simulink model "RotaryPendulum_EV3_SwingUp"  (R2015a)
settings: Solver=ode3  SolverMode=SingleTasking  StartTime=0  StopTime=inf  FixedStep=Ts  RelTol=1e-3
PreLoadFcn:
  | RotaryPendulum_PARAM
InitFcn:
  | simMode = get_param(gcs, 'SimulationMode');
  | if strcmp(simMode, 'external')
  | set_param(gcs,'StopTime', 'Inf');
  | elseif strcmp(simMode, 'normal')
  | set_param(gcs,'StopTime', '10');
  | end
model workspace (MAT data in the model file):
  PulseAmplitude = 200
  Amp = 0
  freq = 0
  Sat = 75
  Ts = 0.008
  threshold = 0.785398163397
  Sig = Simulink.Signal
  Sig.DataType = 'auto'
  Sig.Dimensions = -1
  Sig.DimensionsMode = 'auto'
  Sig.Complexity = 'auto'
  Sig.SampleTime = -1
  Sig.SamplingMode = 'auto'
undefined symbols (not defined in the file): B, C, Center, g, l, m
libraries: simulink x6, legoev3lib x6, simulink_extras x1
settings Model: SimulationMode=external  CovSFcnEnable=off  ExtModeTrigDuration=2  Creator=ngautier  LastModifiedBy=mischak
settings OptimizationCC: EnhancedBackFolding=on  CachingGlobalReferences=on  StrengthReduction=on  OptimizeModelRefInitCode=on  LifeSpan=1
settings DebuggingCC: NonBusSignalsTreatedAsBus=error
settings HardwareCC: ProdLargestAtomicInteger=Long  ProdLargestAtomicFloat=Float  ProdEndianess=LittleEndian  ProdHWDeviceType=ARM Compatible->ARM 9
settings RTWCC: SystemTargetFile=realtime.tlc  GenerateMakefile=off  TemplateMakefile=realtime.tmf  Description=Run on Target Hardware  RTWVerbose=off  IncludeHyperlinkInReport=on
settings ERTTargetCC: CombineOutputUpdateFcns=off  ExtMode=on  ExtModeMexArgs=0 8 9600 30  ERTSrcFileBannerTemplate=realtime_code_template.cgt  ERTHdrFileBannerTemplate=realtime_code_template.cgt  ERTDataSrcFileTemplate=realtime_code_template.cgt  ERTDataHdrFileTemplate=realtime_code_template.cgt  ERTCustomFileTemplate=realtime_file_process.tlc

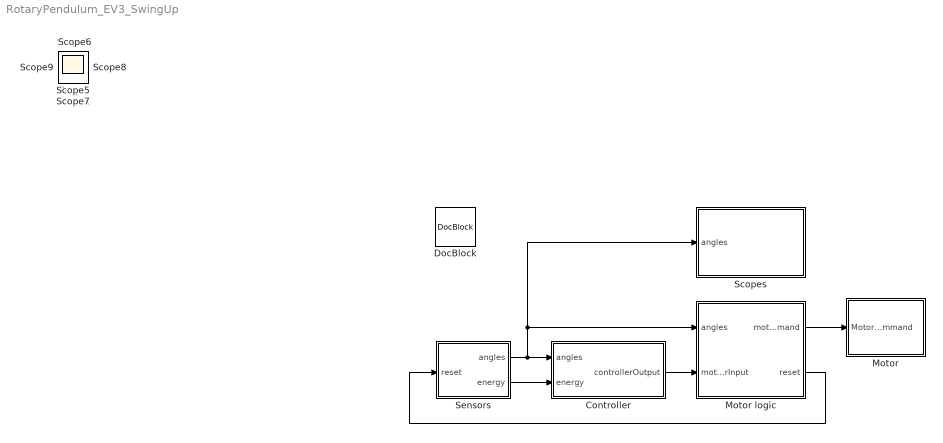
== system RotaryPendulum_EV3_SwingUp ==
  Controller : Subsystem  mask{SUGain=10, outer_gain=[62 9 570 -5], inner_gain=[10 10 370 -10]}
      mask prompts: SUGain "Swing-up amplitude:"; outer_gain "Outer linear gains [al, dal, be, dbe]:"; inner_gain "Inner linear gains [al, dal, be, dbe]:"
      mask TypeOptions SUGain: Swingup controller/Gain
      mask TypeOptions outer_gain: LQR controller/outer_gain
      mask TypeOptions inner_gain: LQR controller/inner_gain
  DocBlock : simulink/Model-Wide Utilities/DocBlock  DocumentType=Text
      content=|
      | Why not use your mobile phone to connect to the EV3?
      |
      | * Enable the portable Wi-Fi hotspot in your mobile phone and note down the
      |   hotspot name and password.
      | * Connect your computer to the hotspot.
      | * Connect the EV3 to the hotspot:
      | ** Navigate to the settings screen (wrench symbol), scroll down and enable [WiFi].
      | ** In the Wi-Fi menu select [Connections] and select the hotspot.
      | ** Enter the hotspot password in [Encryption].
  Motor : Subsystem  mask{sportNumber=C}
      mask prompts: sportNumber "NXT motor port:"
      mask TypeOptions sportNumber: Motor1/sportNumber
      mask Display: image(imread('Motor_icon.jpg'))
  Motor logic : Subsystem  mask{outOfBounds=160}
      mask prompts: outOfBounds "Out of bounds alpha (deg):"
      mask TypeOptions outOfBounds: return&restart/outOfBounds
  Scopes : Subsystem
  Sensors : Subsystem  mask{portNumberAlpha=C, portNumberBeta=B, Value=1}
      mask prompts: portNumberAlpha "NXT alpha sensor port:"; portNumberBeta "NXT beta sensor port:"; Value "Encoder offset (deg):"
      mask TypeOptions portNumberAlpha: Alpha/portNumber
      mask TypeOptions portNumberBeta: Beta/portNumber
      mask TypeOptions Value: Encoder offset/Value
      mask Display: image(imread('Encoders_icon.jpg'))
  Scope{,1..9} (10 alike) : Scope
      Scope1 settings: YMin=3.14159  YMax=3.14159
      Scope2 settings: SaveName=ScopeData2
      Scope3 settings: YMin=3.14159  YMax=3.14159  SaveName=ScopeData3
      Scope4 settings: SaveName=ScopeData4
      Scope5 settings: YMin=0  YMax=0.035  SaveName=ScopeData5
      Scope6 settings: SaveName=ScopeData6
      Scope7 settings: SaveName=ScopeData7
      Scope8 settings: SaveName=ScopeData8
      Scope9 settings: SaveName=ScopeData9
  wires:
  Controller/1(controllerOutput) -> Motor logic/2(motorInput)
  Motor logic/1(motorCommand) -> Motor/1(MotorCommand)
  Sensors/2("energy ") -> Controller/2(energy)
  Sensors/1(angles) -> Motor logic/1(angles), Scopes/1(angles), Controller/1(angles)
  Motor logic/2(reset) -> Sensors/1(reset)

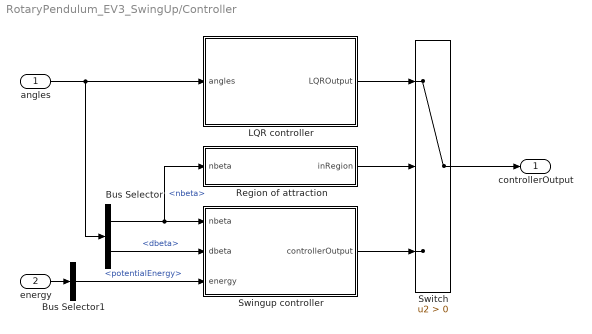
== system RotaryPendulum_EV3_SwingUp/Controller ==
  angles : Inport
  energy : Inport  Port=2
  Bus Selector : BusSelector  OutputSignals=nbeta,dbeta
  Bus Selector1 : BusSelector  OutputSignals=potentialEnergy
  LQR controller : Subsystem  mask{inner_gain=inner_gain, outer_gain=outer_gain}
      mask prompts: inner_gain "Inner gain"; outer_gain "Outer gain"
  Region of attraction : Subsystem  mask{outer_angle=pi/7}
      mask prompts: outer_angle "Simulink:masks:ConstantValue_MP"
      mask TypeOptions outer_angle: Attraction Region/const
      mask Display:
      | %maskValues = get_param(gcb, 'MaskValues');
      | %region = eval(maskValues{1});
      | x = -1:0.1:1;
      | plot(x,abs(x));
      | %ylim([0 2]);
  Swingup controller : Subsystem  SystemSampleTime=Ts  mask{Gain=10}
      mask prompts: Gain "Swing up amplitude"
      mask TypeOptions Gain: Gain1/Gain
      mask Display:
      | maskValues = get_param(gcb, 'MaskValues');
      | fprintf('Swing up gain is: %2.1f %%', eval(maskValues{1}));
  Switch : Switch  Criteria=u2 > Threshold  SampleTime=Ts
  controllerOutput : Outport
  wires:
  energy/1 -> Bus Selector1/1
  Switch/1 -> controllerOutput/1
  Swingup controller/1(controllerOutput) -> Switch/3
  Bus Selector1/1 -> Swingup controller/3(energy)  "<potentialEnergy>"
  Region of attraction/1(inRegion) -> Switch/2
  angles/1 -> Bus Selector/1, LQR controller/1(angles)
  Bus Selector/2 -> Swingup controller/2(dbeta)  "<dbeta>"
  Bus Selector/1 -> Region of attraction/1(nbeta), Swingup controller/1(nbeta)  "<nbeta>"
  LQR controller/1(LQROutput) -> Switch/1

== system RotaryPendulum_EV3_SwingUp/Motor ==
  MotorCommand : Inport
  LimitMotorOutput : Saturate  UpperLimit=100  LowerLimit=-100
  Motor1 : legoev3lib/Motor  sportNumber=C  sstopAction=Brake
  wires:
  MotorCommand/1 -> LimitMotorOutput/1
  LimitMotorOutput/1 -> Motor1/1

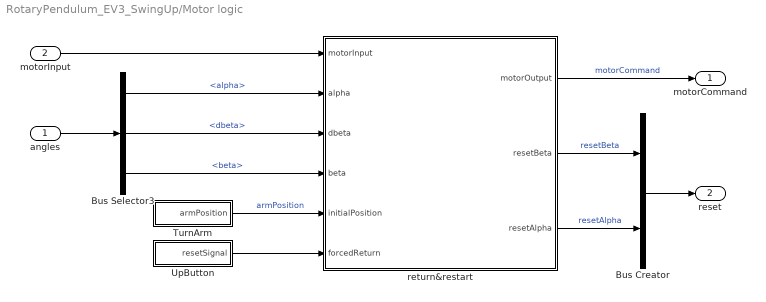
== system RotaryPendulum_EV3_SwingUp/Motor logic ==
  angles : Inport
  motorInput : Inport  Port=2
  Bus Creator : BusCreator  Inputs=2
  Bus Selector3 : BusSelector  OutputSignals=alpha,dbeta,beta
  TurnArm : Subsystem
  UpButton : Subsystem  mask{buttonType=Center}
      mask prompts: buttonType "Button:"
      mask TypeOptions buttonType: Center button/buttonType
  return&restart : Stateflow chart  TreatAsAtomicUnit=on  mask{outOfBounds=outOfBounds}
      mask prompts: outOfBounds "Out of bounds position"
  motorCommand : Outport
  reset : Outport  Port=2
  wires:
  return&restart/3(resetAlpha) -> Bus Creator/2  "resetAlpha"
  return&restart/1(motorOutput) -> motorCommand/1  "motorCommand"
  return&restart/2(resetBeta) -> Bus Creator/1  "resetBeta"
  motorInput/1 -> return&restart/1(motorInput)
  angles/1 -> Bus Selector3/1
  Bus Selector3/1 -> return&restart/2(alpha)  "<alpha>"
  UpButton/1("resetSignal ") -> return&restart/6(forcedReturn)
  Bus Selector3/2 -> return&restart/3(dbeta)  "<dbeta>"
  Bus Selector3/3 -> return&restart/4(beta)  "<beta>"
  TurnArm/1(armPosition) -> return&restart/5(initialPosition)  "armPosition"
  Bus Creator/1 -> reset/1

== system RotaryPendulum_EV3_SwingUp/Scopes ==
  angles : Inport
  Bus Selector : BusSelector  OutputSignals=alpha,nbeta,dalpha,dbeta
  Scope : Scope  NumInputPorts=4
      settings: TimeRange=10  YMin=-0.475~-0.02~-3~-12.5  YMax=0~0.035~10~17.5  SaveName=ScopeData10
  wires:
  Bus Selector/2 -> Scope/2  "<nbeta>"
  Bus Selector/4 -> Scope/4  "<dbeta>"
  Bus Selector/3 -> Scope/3  "<dalpha>"
  Bus Selector/1 -> Scope/1  "<alpha>"
  angles/1 -> Bus Selector/1

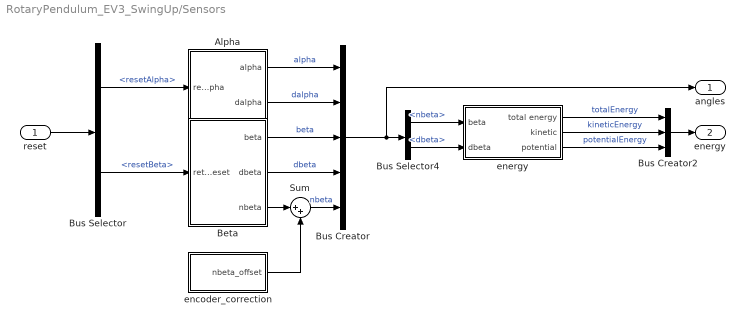
== system RotaryPendulum_EV3_SwingUp/Sensors ==
  reset : Inport
  Alpha : Subsystem  mask{portNumber=C}
      mask prompts: portNumber "NXT brick output port:"
      mask TypeOptions portNumber: AlphaEncoder/portNumber
      mask Display: disp('\alpha, d_t \alpha', 'texmode','on')
  Beta : Subsystem  mask{portNumber=B}
      mask prompts: portNumber "NXT brick output port:"
      mask TypeOptions portNumber: BetaEncoder/portNumber
      mask Display: disp('\beta, d_t \beta', 'texmode','on')
  Bus Creator : BusCreator  Inputs=5
  Bus Creator2 : BusCreator  Inputs=3
  Bus Selector : BusSelector  OutputSignals=resetAlpha,resetBeta
  Bus Selector4 : BusSelector  OutputSignals=nbeta,dbeta
  Sum : Sum  Inputs=|++
  encoder_correction : Subsystem
  energy : Subsystem
  angles : Outport
  "energy " : Outport  Port=2
  wires:
  Bus Creator/1 -> angles/1, Bus Selector4/1
  Beta/1(beta) -> Bus Creator/3  "beta"
  Beta/2(dbeta) -> Bus Creator/4  "dbeta"
  Beta/3(nbeta) -> Sum/1
  Bus Creator2/1 -> "energy "/1
  Alpha/2(dalpha) -> Bus Creator/2  "dalpha"
  Bus Selector/2 -> Beta/1(returnReset)  "<resetBeta>"
  energy/1(total energy) -> Bus Creator2/1  "totalEnergy"
  energy/2(kinetic) -> Bus Creator2/2  "kineticEnergy"
  Alpha/1(alpha) -> Bus Creator/1  "alpha"
  energy/3(potential) -> Bus Creator2/3  "potentialEnergy"
  Bus Selector4/1 -> energy/1(beta)  "<nbeta>"
  Bus Selector4/2 -> energy/2(dbeta)  "<dbeta>"
  Sum/1 -> Bus Creator/5  "nbeta"
  reset/1 -> Bus Selector/1
  Bus Selector/1 -> Alpha/1(resetAlpha)  "<resetAlpha>"
  encoder_correction/1(nbeta_offset) -> Sum/2

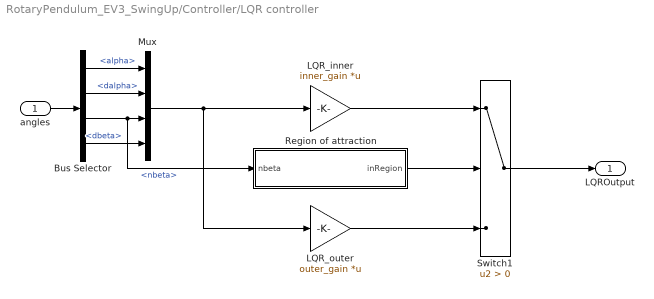
== system RotaryPendulum_EV3_SwingUp/Controller/LQR controller ==
  angles : Inport
  Bus Selector : BusSelector  OutputSignals=alpha,dalpha,nbeta,dbeta
  LQR_inner : Gain  Gain=inner_gain  Multiplication=Matrix(K*u)
  LQR_outer : Gain  Gain=outer_gain  Multiplication=Matrix(K*u)
  Mux : Mux
  Region of attraction : Subsystem  mask{const=2.5*pi/180}
      mask prompts: const "Simulink:masks:ConstantValue_MP"
      mask TypeOptions const: Attraction Region/const
      mask Display:
      | %maskValues = get_param(gcb, 'MaskValues');
      | %region = eval(maskValues{1});
      | x = -1:0.1:1;
      | plot(x,abs(x));
      | %ylim([0 2]);
  Switch1 : Switch  Criteria=u2 > Threshold  SampleTime=Ts
  LQROutput : Outport
  wires:
  Switch1/1 -> LQROutput/1
  LQR_outer/1 -> Switch1/3
  Region of attraction/1(inRegion) -> Switch1/2
  LQR_inner/1 -> Switch1/1
  Bus Selector/1 -> Mux/1  "<alpha>"
  Bus Selector/2 -> Mux/2  "<dalpha>"
  Bus Selector/3 -> Region of attraction/1(nbeta), Mux/3  "<nbeta>"
  Bus Selector/4 -> Mux/4  "<dbeta>"
  angles/1 -> Bus Selector/1
  Mux/1 -> LQR_outer/1, LQR_inner/1

== system RotaryPendulum_EV3_SwingUp/Controller/Region of attraction ==
  nbeta : Inport
  Abs : Abs
  Attraction Region : simulink/Logic and Bit Operations/Compare To Constant  relop=<=  const=outer_angle  OutDataTypeStr=boolean
  inRegion : Outport
  wires:
  nbeta/1 -> Abs/1
  Abs/1 -> Attraction Region/1
  Attraction Region/1 -> inRegion/1

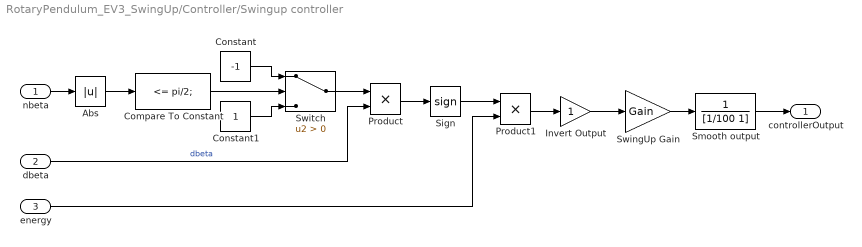
== system RotaryPendulum_EV3_SwingUp/Controller/Swingup controller ==
  nbeta : Inport
  dbeta : Inport  Port=2
  energy : Inport  Port=3
  Abs : Abs
  Compare To Constant : simulink/Logic and Bit Operations/Compare To Constant  relop=<=  const=pi/2;  OutDataTypeStr=boolean
  Constant : Constant  Value=-1
  Constant1 : Constant
  Invert Output : Gain
  Product : Product
  Product1 : Product
  Sign : Signum  SampleTime=Ts
  Smooth output : TransferFcn  Denominator=[1/100 1]
  SwingUp Gain : Gain  Gain=Gain
  Switch : Switch  Criteria=u2 > Threshold
  controllerOutput : Outport
  wires:
  dbeta/1 -> Product/2  "dbeta"
  SwingUp Gain/1 -> Smooth output/1
  Product/1 -> Sign/1
  nbeta/1 -> Abs/1
  Product1/1 -> Invert Output/1
  Smooth output/1 -> controllerOutput/1
  Switch/1 -> Product/1
  Compare To Constant/1 -> Switch/2
  Constant/1 -> Switch/1
  Constant1/1 -> Switch/3
  Abs/1 -> Compare To Constant/1
  Invert Output/1 -> SwingUp Gain/1
  Sign/1 -> Product1/1
  energy/1 -> Product1/2

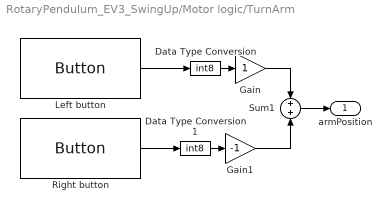
== system RotaryPendulum_EV3_SwingUp/Motor logic/TurnArm ==
  Data Type Conversion : DataTypeConversion  OutDataTypeStr=int8
  Data Type Conversion1 : DataTypeConversion  OutDataTypeStr=int8
  Gain : Gain  OutDataTypeStr=int8  SampleTime=Ts
  Gain1 : Gain  Gain=-1  OutDataTypeStr=int8  SampleTime=Ts
  Left button : legoev3lib/Button  buttonType=Left  sampleTime=Ts
  Right button : legoev3lib/Button  buttonType=Right  sampleTime=Ts
  Sum1 : Sum  Inputs=+|+
  armPosition : Outport
  wires:
  Sum1/1 -> armPosition/1
  Left button/1 -> Data Type Conversion/1
  Right button/1 -> Data Type Conversion1/1
  Gain/1 -> Sum1/1
  Gain1/1 -> Sum1/2
  Data Type Conversion/1 -> Gain/1
  Data Type Conversion1/1 -> Gain1/1

== system RotaryPendulum_EV3_SwingUp/Motor logic/UpButton ==
  Center button : legoev3lib/Button  buttonType=Center  sampleTime=Ts
  Data Type Conversion : DataTypeConversion  OutDataTypeStr=boolean  SampleTime=Ts
  "resetSignal " : Outport
  wires:
  Center button/1 -> Data Type Conversion/1
  Data Type Conversion/1 -> "resetSignal "/1  "resetSignal"

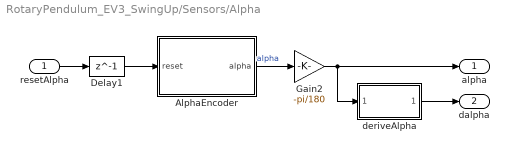
== system RotaryPendulum_EV3_SwingUp/Sensors/Alpha ==
  resetAlpha : Inport
  AlphaEncoder : Subsystem  mask{portNumber=C}
      mask prompts: portNumber "NXT brick output port:"
      mask TypeOptions portNumber: Encoder/portNumber
      mask Display:
      | port = get_param(gcb,'MaskValues');
      | fprintf(['Encoder port is: ' port{1}]);
  Delay1 : Delay  DelayLength=1
  Gain2 : Gain  Gain=-pi/180
  deriveAlpha : Subsystem
  alpha : Outport
  dalpha : Outport  Port=2
  wires:
  Gain2/1 -> alpha/1, deriveAlpha/1(alpha)
  AlphaEncoder/1("alpha ") -> Gain2/1  "alpha"
  deriveAlpha/1(dalpha) -> dalpha/1
  resetAlpha/1 -> Delay1/1
  Delay1/1 -> AlphaEncoder/1(reset)

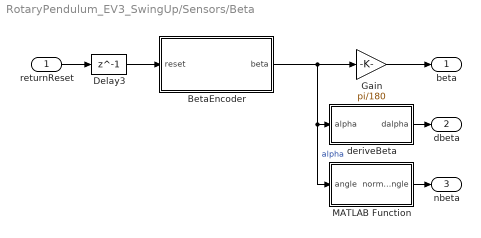
== system RotaryPendulum_EV3_SwingUp/Sensors/Beta ==
  returnReset : Inport
  BetaEncoder : Subsystem  mask{portNumber=B}
      mask prompts: portNumber "NXT brick output port:"
      mask TypeOptions portNumber: Encoder1/portNumber
      mask Display:
      | port = get_param(gcb,'MaskValues');
      | fprintf(['Encoder port is: ' port{1}]);
  Delay3 : Delay  DelayLength=1  InitialCondition=0
  Gain : Gain  Gain=pi/180
  MATLAB Function : MATLAB Function  TreatAsAtomicUnit=on
  deriveBeta : Subsystem
  beta : Outport
  dbeta : Outport  Port=2
  nbeta : Outport  Port=3
  wires:
  MATLAB Function/1(normalizedAngle) -> nbeta/1
  deriveBeta/1(dalpha) -> dbeta/1
  returnReset/1 -> Delay3/1
  Delay3/1 -> BetaEncoder/1(reset)
  BetaEncoder/1("beta ") -> Gain/1, deriveBeta/1(alpha), MATLAB Function/1(angle)  "alpha"
  Gain/1 -> beta/1

== system RotaryPendulum_EV3_SwingUp/Sensors/encoder_correction ==
  Degrees to Radians : simulink_extras/Transformations/Degrees to Radians
  Encoder offset : Constant  Value=Value
  nbeta_offset : Outport
  wires:
  Encoder offset/1 -> Degrees to Radians/1
  Degrees to Radians/1 -> nbeta_offset/1

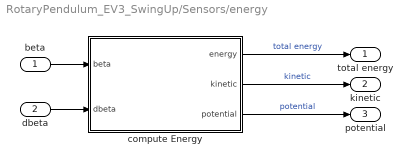
== system RotaryPendulum_EV3_SwingUp/Sensors/energy ==
  beta : Inport
  dbeta : Inport  Port=2
  compute Energy : MATLAB Function  TreatAsAtomicUnit=on
  total energy : Outport
  kinetic : Outport  Port=2
  potential : Outport  Port=3
  wires:
  compute Energy/1(energy) -> total energy/1  "total energy"
  beta/1 -> compute Energy/1(beta)
  compute Energy/3(potential) -> potential/1  "potential"
  dbeta/1 -> compute Energy/2(dbeta)
  compute Energy/2(kinetic) -> kinetic/1  "kinetic"

== system RotaryPendulum_EV3_SwingUp/Controller/LQR controller/Region of attraction ==
  nbeta : Inport
  Abs : Abs
  Attraction Region : simulink/Logic and Bit Operations/Compare To Constant  relop=<=  const=const  OutDataTypeStr=boolean
  inRegion : Outport
  wires:
  Attraction Region/1 -> inRegion/1
  Abs/1 -> Attraction Region/1
  nbeta/1 -> Abs/1

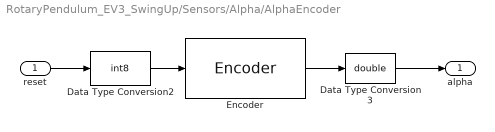
== system RotaryPendulum_EV3_SwingUp/Sensors/Alpha/AlphaEncoder ==
  reset : Inport
  Data Type Conversion2 : DataTypeConversion  OutMin=0  OutDataTypeStr=int8
  Data Type Conversion3 : DataTypeConversion  OutDataTypeStr=double
  Encoder : legoev3lib/Encoder  portNumber=C  opMode=Reset by external signal  sampleTime=Ts
  "alpha " : Outport
  wires:
  Data Type Conversion3/1 -> "alpha "/1
  reset/1 -> Data Type Conversion2/1
  Encoder/1 -> Data Type Conversion3/1
  Data Type Conversion2/1 -> Encoder/1

== system RotaryPendulum_EV3_SwingUp/Sensors/Alpha/deriveAlpha ==
  alpha : Inport
  Discrete Derivative1 : simulink/Discrete/Discrete Derivative  gainval=1.0  ICPrevScaledInput=0.0  InputProcessing=Inherited  OutMin=[]  OutMax=[]  OutDataType=fixdt(1, 16)  OutScaling=2^-10  DoSatur=off
  Transfer Fcn : TransferFcn  Denominator=[1/50 1]
  Transfer Fcn1 : TransferFcn  Denominator=[1/20 1]
  dalpha : Outport
  wires:
  Transfer Fcn1/1 -> dalpha/1
  alpha/1 -> Transfer Fcn/1
  Transfer Fcn/1 -> Discrete Derivative1/1
  Discrete Derivative1/1 -> Transfer Fcn1/1

== system RotaryPendulum_EV3_SwingUp/Sensors/Beta/BetaEncoder ==
  reset : Inport
  Data Type Conversion : DataTypeConversion  OutDataTypeStr=double
  Data Type Conversion1 : DataTypeConversion  OutMin=0  OutDataTypeStr=int8
  Encoder1 : legoev3lib/Encoder  portNumber=B  opMode=Reset by external signal  sampleTime=Ts
  "beta " : Outport
  wires:
  Data Type Conversion1/1 -> Encoder1/1
  reset/1 -> Data Type Conversion1/1
  Encoder1/1 -> Data Type Conversion/1  "beta"
  Data Type Conversion/1 -> "beta "/1

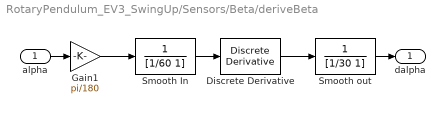
== system RotaryPendulum_EV3_SwingUp/Sensors/Beta/deriveBeta ==
  alpha : Inport
  Discrete Derivative : simulink/Discrete/Discrete Derivative  gainval=1.0  ICPrevScaledInput=0.0  InputProcessing=Inherited  OutMin=[]  OutMax=[]  OutDataType=fixdt(1, 16)  OutScaling=2^-10  DoSatur=off
  Gain1 : Gain  Gain=pi/180
  Smooth In : TransferFcn  Denominator=[1/60 1]
  Smooth out : TransferFcn  Denominator=[1/30 1]
  dalpha : Outport
  wires:
  alpha/1 -> Gain1/1
  Smooth out/1 -> dalpha/1
  Gain1/1 -> Smooth In/1
  Smooth In/1 -> Discrete Derivative/1
  Discrete Derivative/1 -> Smooth out/1

== stateflow chart RotaryPendulum_EV3_SwingUp/Motor logic/return&restart ==
  state normalPosition
    state NormalMode
      du:motorOutput = motorInput;
    state Start
      motorOutput = amplitude * sin(2*pi*frequency*time);
      resetBeta = 0;
    state ReturnToInitialPosition
      en: resetAlpha = 0;
      du: motorOutput = - (alpha)/abs(alpha)*returnSpeed;
      exit: motorOutput = 0;
    state Stabilize
      exit: resetBeta = 1;
    Start -> NormalMode [order 1] : [time > startDuration]
    NormalMode -> ReturnToInitialPosition : [abs(alpha) > outOfBounds*pi/180 || forcedReturn || abs(beta) > 2*pi]
    Start -> Start [order 2] : after(0.05,sec){time+=0.05;}
    Stabilize -> Start [order 1] : [counter > 20]{time = 0;}
    ReturnToInitialPosition -> Stabilize : [abs(alpha) < threshold_alpha]{counter = 0;}
    Stabilize -> Stabilize [order 2] : after(0.1,sec)[abs(dbeta) < threshold_beta]{counter++;}
  state changeInitialPos
    ex: resetAlpha =1;
  (default) -> NormalMode [order 2]
  (default) -> Start [order 1] : [counter <0] { time=0}
  changeInitialPos -> changeInitialPos [order 3] : [initialPosition > 0]{motorOutput = -returnSpeed;}
  normalPosition -> changeInitialPos : [abs(initialPosition) > 0]
  changeInitialPos -> changeInitialPos [order 1] : [initialPosition < 0]{motorOutput = returnSpeed;}
  changeInitialPos -> ReturnToInitialPosition [order 2] : after(.05,sec)[initialPosition == 0]
  data: motorInput input size=1; alpha input size=1; motorOutput output double size=1; outOfBounds parameter double size=1; returnSpeed constant double size=1 =10; threshold_beta constant double size=1 =0.002; dbeta input double; counter local int32 size=1 =-1; resetBeta output double; startDuration constant double =.5; beta input size=1; initialPosition input size=1; forcedReturn input boolean size=1; resetAlpha output double; frequency constant double =2; time local double; amplitude constant double =10; pi constant double =pi; threshold_alpha constant double =0.0005

== matlab function RotaryPendulum_EV3_SwingUp/Sensors/energy/compute Energy ==
  data: beta input; energy output; dbeta input; l parameter; m parameter; g parameter; kinetic output; potential output
function [energy, kinetic, potential] = computeEnergy(beta,dbeta,l,m,g)
%#codegen 

kinetic   = 1/2*1/3*m*l^2*dbeta^2/(m*g*l);
potential = m*g*l*(cos(beta) - 1)/(m*g*l);
energy    = kinetic + potential;

== matlab function RotaryPendulum_EV3_SwingUp/Sensors/Beta/MATLAB Function ==
  data: angle input; normalizedAngle output size=1
function normalizedAngle = fcn(angle)
%#codegen
if angle == 0;
    normalizedAngle = pi;
else
    sgn = sign(angle);
    angle = sgn*mod(abs(angle),360);
    normalizedAngle = sgn*(pi - abs(angle)*pi/180);
end
